simulink model "s32ze_dio_FreeMASTER"  (R2024a)
settings: Solver=FixedStepAuto  StartTime=0.0  StopTime=10.0  FixedStep=1  RelTol=1e-3  EnableMultiTasking=on
PreLoadFcn:
  | % NXP_MBDT_S32ZE callback: DO NOT REMOVE
  | mbd_s32ze.common.nxp.model_callbacks.preLoadFcn();
PostLoadFcn:
  | % NXP_MBDT_S32ZE callback: DO NOT REMOVE
  | mbd_s32ze.common.nxp.model_callbacks.postLoadFcn();
InitFcn:
  | % NXP_MBDT_S32ZE callback: DO NOT REMOVE
  | mbd_s32ze.common.nxp.model_callbacks.initFcn();
libraries: mbd_s32ze_utility_library x2, mbd_s32ze_io_library x1
Description:
  | Dio EBT
  | 
  | 
  | 
  |         Dio EBT
  |         <a href="matlab:open(fullfile(mbd_find_s32ze_root(),'S32ZE_Examples\r52\dio\s32ze_dio_ebt\s32ze_dio_ebt.mdl'))">Open Example
  |         The s32ze_dio_ebt.mdl example shows how to use DIO FilpChannel functionality.
  | 
  |             After the application is deployed on target, the D12 LED should toggle every 1 second. The versionInfo variable stores the version information of this module, including module id, vendor id and vendor specific version numbers.
  | 
  |             Note: the initialization settings for the components used in this example represent just a default EB Tresos available configuration. Users can change the configuration of the application to fit special requirements.
  | 
  |         Toolchain Supported
  | 
  | 
  |                 S32 Design Studio v3.5.13
  | 
  | 
  |         Required Hardware
  | 
  | 
  |                 Personal Computer
  | 
  |                 S32Z2xx/S32E2xx
  | 
  |                 12V Power Supply
  | 
  |                 Micro USB cable
  | 
  |                 S32 Debugger probe
  | 
  | 
  |         Prepare the Demo
  | 
  | 
  |                 Open the model and select the processor package. This model is configured for the S32E2xx-bga975 hardware package. If you would like to change the processor package, please follow the steps described in the Customization Options section.
  | 
  |                 Connect the S32 Debugger probe to the J129 JTAG pin connector on the EVB.
  | 
  |                 Build and Download the program on the target processor.
  | 
  | 
  |         Running the Demo
  | 
  | 
  |                 The D12 LED should toggle every 1 seconds.
  | 
  | 
  |         Customization Options
  | 
  | 
  |                 How to change the processor package - visit section 6.8 of <a href="matlab:web(fullfile(mbd_find_s32ze_root(), 'mbdtbx_s32ze', 'help', 'release_notes.html'), '-browser')">Model_Based_Design_Toolbox_S32ZE_Series_Release_Notes
  | 
  |                 How to create a configuration project for a custom board - visit section 6.6 of <a href="matlab:web(fullfile(mbd_find_s32ze_root(), 'mbdtbx_s32ze', 'help', 'release_notes.html'), '-browser')">Model_Based_Design_Toolbox_S32ZE_Series_Release_Notes
  | 
  |                 For S32Z and S32E Design Tools and Files, please visit <a href="https://www.nxp.com/products/processors-and-microcontrollers/s32-automotive-platform/s32z-and-s32e-real-time-processors:S32Z-E-REAL-TIME-PROCESSORS">S32ZE Microcontrollers
settings Model: DataDictionary=s32ze_dio_FreeMASTER.sldd  Creator=nxa06644  LastModifiedBy=nxf90129
settings SolverCC: AlgebraicLoopSolver=TrustRegion
settings OptimizationCC: EnhancedBackFolding=on  PassReuseOutputArgsAs=Individual arguments  MaxStackSize=64  OptimizeBlockOrder=speed  DifferentSizesBufferReuse=on  OptimizationCustomize=off  EfficientTunableParamExpr=on
settings DebuggingCC: InheritedTsInSrcMsg=none  ParameterTunabilityLossMsg=error  UnconnectedInputMsg=warning  UnconnectedOutputMsg=warning  UnconnectedLineMsg=warning
settings HardwareCC: ProdBitPerPointer=32  ProdBitPerSizeT=32  ProdBitPerPtrDiffT=32  ProdLargestAtomicInteger=Long  ProdLargestAtomicFloat=Double  ProdWordSize=32  ProdHWDeviceType=ARM Compatible->ARM Cortex
settings ModelReferenceCC: EnableRefExpFcnMdlSchedulingChecks=on
settings SFSimCC: MATLABDynamicMemAlloc=off  CustomCodeUndefinedFunction=UseInterfaceOnly
settings RTWCC: Description=Embedded Coder  SystemTargetFile=ert.tlc  HardwareBoard=NXP S32ZE2xx  TemplateMakefile=ert_default_tmf  GenerateReport=on  Toolchain=NXP S32 Design Studio GCC (S32ZE)  BuildConfiguration=Faster Runs  IncludeHyperlinkInReport=on  LaunchReport=on  GenerateTraceInfo=on  GenerateTraceReport=on  GenerateTraceReportSl=on  GenerateTraceReportSf=on  GenerateTraceReportEml=on  GPUComputeCapability=3.5  DLArmComputeVersion=19.05
settings CodeAppCC: ForceParamTrailComments=on  IgnoreCustomStorageClasses=off  OperatorAnnotations=on  SimulinkDataObjDesc=on  SFDataObjDesc=on  InsertBlockDesc=on
settings ERTTargetCC: ERTSrcFileBannerTemplate=mbd_s32ze_ert_code_template.cgt  ERTHdrFileBannerTemplate=mbd_s32ze_ert_code_template.cgt  ERTDataSrcFileTemplate=mbd_s32ze_ert_code_template.cgt  ERTDataHdrFileTemplate=mbd_s32ze_ert_code_template.cgt

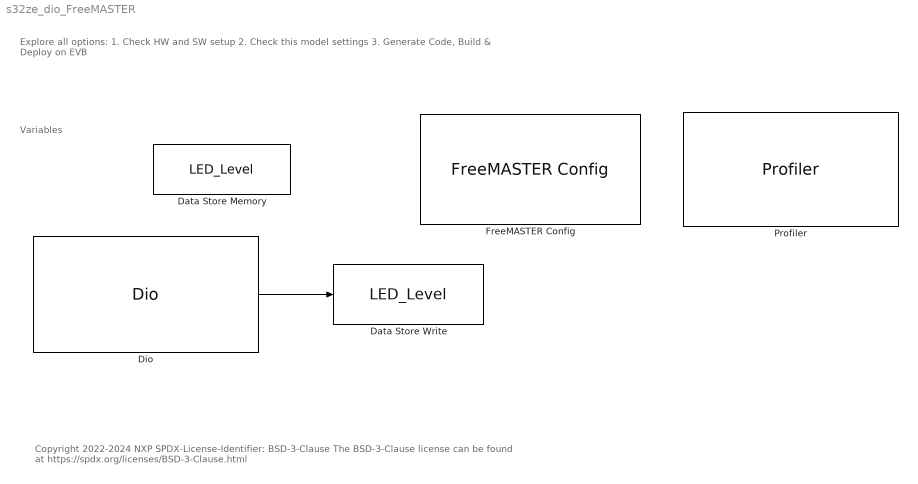
== system s32ze_dio_FreeMASTER ==
  note: Variables
  note: Explore all options:
      | 1. Check HW and SW setup
      | 2. Check this model settings
      | 3. Generate Code, Build & Deploy on EVB
  note: Copyright 2022-2024 NXP
      |
      | SPDX-License-Identifier: BSD-3-Clause
      | The BSD-3-Clause license can be found at https://spdx.org/licenses/BSD-3-Clause.html
  Data Store Memory : DataStoreMemory  DataStoreName=LED_Level  WriteAfterWriteMsg=warning  ShowAdditionalParam=off
  Data Store Write : DataStoreWrite  DataStoreName=LED_Level  IndexOptions=Index vector (dialog)  Indices=1  OutputSizes=1
  Dio : mbd_s32ze_io_library/Dio  api_func=Dio_FlipChannel  channel=RED_D12_LED  channel_group=No channel groups configured  port=DioPort_0  gpioSim=off  text=<binary blob, 1229 chars, not shown>
  FreeMASTER Config : mbd_s32ze_utility_library/FreeMASTER Blocks/FreeMASTER Config  connection_type=Serial  instance=LinflexD_9  baudrate=115200  isr_prio=5  cantxid=0x7aa  cantxidext=on  cantxobj=5  canrxid=0x7aa  canrxidext=on  canrxobj=5  mode=Short Interrupt  scope_use=1  scope_max_vars=8  automatic_buff_size=on  buff_size=255  default_rfifo_size=on  rfifo_size=32
  Profiler : mbd_s32ze_utility_library/Profiler Blocks/Profiler  index=0  timerName=Cortex-R52 PMU  getUnit=Ticks
  wires:
  Dio/1 -> Data Store Write/1
